simulink model "test_downshift"  (Simulink 7.3)
settings: Solver=ode45  StartTime=0  StopTime=500  RelTol=1e-3
libraries: xbsIndex_r4 x7, simulink x2, isi_correlator_lib x1
settings Model: Creator=wjm  LastModifiedBy=wjm

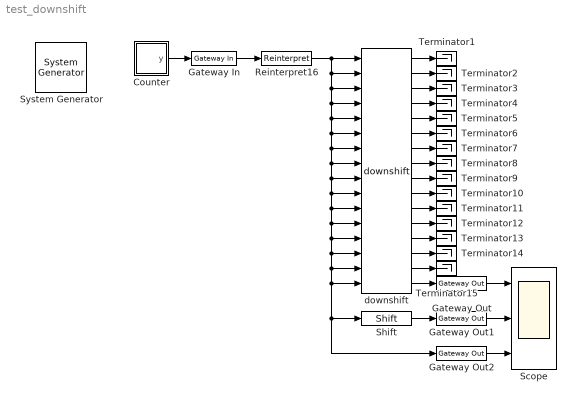
== system test_downshift ==
  " System Generator" : xbsIndex_r4/ System Generator  Tag=genX  SystemSampleTime=-1  xilinxfamily=Virtex6  part=xc6vsx315t  speed=-3  package=ff1156  synthesis_tool=XST  clock_wrapper=Clock Enables  directory=./netlist  testbench=off  simulink_period=1  sysclk_period=10  dcm_input_clock_period=10  incr_netlist=off  trim_vbits=Everywhere in SubSystem  dbl_ovrd=According to Block Masks  core_generation=According to Block Masks  run_coregen=off  deprecated_control=off  eval_field=0  block_type=sysgen
      settings: block_version=11.3
  Counter : Subsystem  AncestorBlock=simulink/Sources/Counter Free-Running  mask(Counter Free-Running){NumBits=8, tsamp=1}
      mask prompts: NumBits "Number of Bits"; tsamp "Sample time:"
      mask help: This block is a free-running counter that overflows back to zero after it has reached the maximum value possible for the specified number of bits. The count is always initialized to zero. The output is normally an unsigned integer with the specified number of bits.
      mask Display: plot( 0.05+0.9/8*[0 1 1 2 2 3 3 4 4 5 5 6 6 7 7 8 8], 0.3+0.65/3*[0 0 1 1 2 2 3 3 0 0 1 1 2 2 3 3 0] )
  Gateway In : xbsIndex_r4/Gateway In  arith_type=Unsigned  n_bits=8  bin_pt=0  quantization="Round  (unbiased: +/- Inf)"  overflow=Saturate  period=1  dbl_ovrd=off  timing_constraint=None  locs_specified=off  LOCs={}  block_type=gatewayin
      settings: infoedit="Gateway in block.  Converts inputs of type Simulink integer, double and fixed point to  Xilinx fixed point type.<br><br>Hardware notes:  In hardware these blocks become top level input ports."  block_version=11.3
  Gateway Out : xbsIndex_r4/Gateway Out  hdl_port=on  timing_constraint=None  locs_specified=off  LOCs={}  block_type=gatewayout
      settings: infoedit="Gateway out block.  Converts Xilinx fixed point inputs into ouputs of type Simulink integer, double, or fixed point.<br><br>Hardware notes:  In hardware these blocks become top level output ports or are discarded, depending on how they are configured."  block_version=11.3
  Gateway Out1 : xbsIndex_r4/Gateway Out  hdl_port=on  timing_constraint=None  locs_specified=off  LOCs={}  block_type=gatewayout
      settings: infoedit="Gateway out block.  Converts Xilinx fixed point inputs into ouputs of type Simulink integer, double, or fixed point.<br><br>Hardware notes:  In hardware these blocks become top level output ports or are discarded, depending on how they are configured."  block_version=11.3
  Gateway Out2 : xbsIndex_r4/Gateway Out  hdl_port=on  timing_constraint=None  locs_specified=off  LOCs={}  block_type=gatewayout
      settings: infoedit="Gateway out block.  Converts Xilinx fixed point inputs into ouputs of type Simulink integer, double, or fixed point.<br><br>Hardware notes:  In hardware these blocks become top level output ports or are discarded, depending on how they are configured."  block_version=11.3
  Reinterpret16 : xbsIndex_r4/Reinterpret  force_arith_type=on  arith_type="Signed  (2's comp)"  force_bin_pt=on  bin_pt=7  block_type=reinterpret
      settings: infoedit="Changes signal type without altering the binary representation.   You can changed the signal between signed and unsigned, and relocate the binary point.<br><br>Hardware notes: In hardware this block costs nothing.<br><br>Example:  Suppose the input is 6 bits wide, signed, with 2 fractional bits, and the output is forced to unsigned with 0 fractional bits.  Then an input of -2.0 (1110.00 in binary 2's complement) becomes an output of 56 (111000 in binary)."  block_version=11.3
  Scope : Scope  NumInputPorts=3
      settings: YMin=-5~-5~-5  YMax=5~5~5
  Shift : xbsIndex_r4/Shift  shift_dir=Right  shift_bits=1  en=off  latency=0  precision=Full  arith_type="Signed  (2's comp)"  n_bits=16  bin_pt=14  quantization=Truncate  overflow=Wrap  dbl_ovrd=off  block_type=shift
      settings: block_version=11.3
  Terminator{1..15} (15 alike) : Terminator
  downshift : isi_correlator_lib/downshift  SystemSampleTime=-1  bit_width=8
  wires:
  downshift/1 -> Terminator1/1
  downshift/2 -> Terminator2/1
  downshift/3 -> Terminator3/1
  downshift/4 -> Terminator4/1
  downshift/5 -> Terminator5/1
  downshift/6 -> Terminator6/1
  downshift/7 -> Terminator7/1
  downshift/8 -> Terminator8/1
  downshift/9 -> Terminator9/1
  downshift/10 -> Terminator10/1
  downshift/11 -> Terminator11/1
  downshift/12 -> Terminator12/1
  downshift/13 -> Terminator13/1
  downshift/14 -> Terminator14/1
  downshift/15 -> Terminator15/1
  downshift/16 -> Gateway Out/1
  Gateway In/1 -> Reinterpret16/1
  Counter/1(y) -> Gateway In/1
  Gateway Out/1 -> Scope/1
  Shift/1 -> Gateway Out1/1
  Gateway Out1/1 -> Scope/2
  Gateway Out2/1 -> Scope/3
  Reinterpret16/1 -> downshift/1, downshift/2, downshift/3, downshift/4, downshift/5, downshift/6, downshift/7, downshift/8, downshift/9, downshift/10, downshift/11, downshift/12, downshift/13, downshift/14, downshift/15, downshift/16, Shift/1, Gateway Out2/1

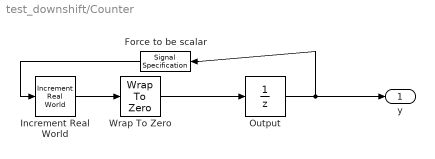
== system test_downshift/Counter ==
  Force to be scalar : SignalSpecification  DisableCoverage=on  Dimensions=1  OutDataType=fixdt(1, 16)  OutScaling=2^0
  Increment Real World : simulink/Additional Math & Discrete/Additional Math: Increment - Decrement/Increment Real World  DisableCoverage=on  SystemSampleTime=-1
  Output : UnitDelay  X0=0.0  SampleTime=tsamp
  Wrap To Zero : simulink/Discontinuities/Wrap To Zero  DisableCoverage=on  SystemSampleTime=-1  Threshold=(2^(NumBits))-1
  y : Outport  OutDataType=fixdt(1, 16)  OutScaling=2^0
  wires:
  Output/1 -> y/1, Force to be scalar/1
  Increment Real World/1 -> Wrap To Zero/1
  Wrap To Zero/1 -> Output/1
  Force to be scalar/1 -> Increment Real World/1
